simulink model "c2_non_lineare"  (R2021a)
settings: Solver=VariableStepAuto  StartTime=0.0  StopTime=10.0  RelTol=1e-3
values from neighbouring files (symbols this model uses):
  beta = 1.3    [c2.m]
  DD = 8    [c2.m]
  delta_1 = 3*10^4    (= 30000)    [c2.m]
  delta_2 = 0.2    [c2.m]
  delta_3 = 0.02    [c2.m]
  gamma_1 = 0.75    [c2.m]
  gamma_2 = 0.15    [c2.m]
  J = 20    [c2.m]
  phi = 0.04    [c2.m]
  RR_s = mu_s / G_0    [c2.m]
  u_e = (acos(-(gamma_2/gamma_1)*30*8e-4+1)+phi)/beta    [c2.m]
  x_1e = (delta_2 * x_2e + delta_3*x_2e^2) / delta_1    (= 0.0008)    [c2.m]
  x_2e = omega_e    (= 30)    [c2.m]
undefined symbols (not defined in the file or in its folder): NN, omega_d, omega_n, R_d
libraries: cstblocks x1
settings Model: Creator=lucac  LastModifiedBy=lucac

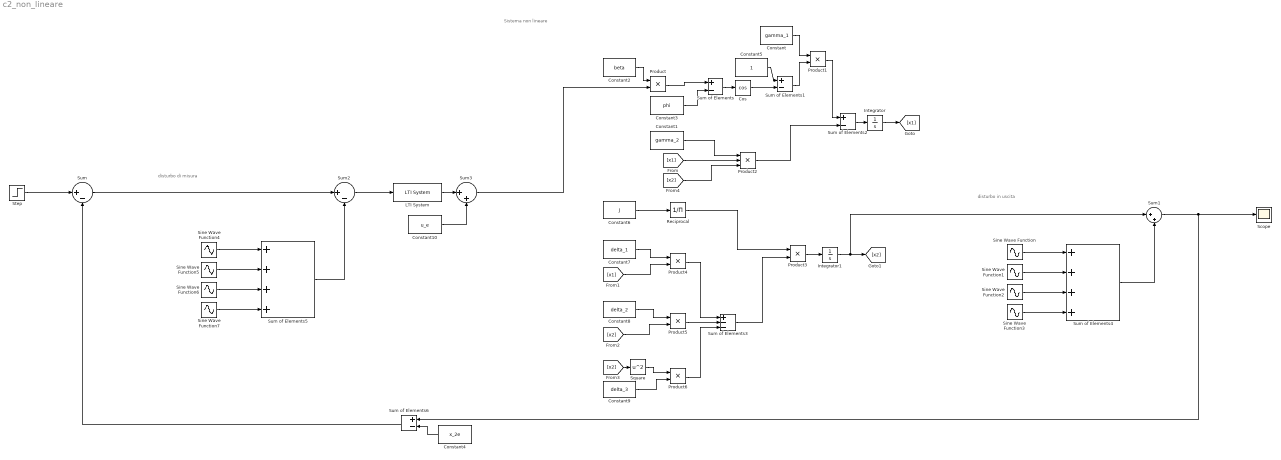
== system c2_non_lineare ==
  note: Sistema non lineare
  note: disturbo di misura
  note: disturbo in uscita
  Constant : Constant  Value=gamma_1
  Constant1 : Constant  Value=gamma_2
  Constant10 : Constant  Value=u_e
  Constant2 : Constant  Value=beta
  Constant3 : Constant  Value=phi
  Constant4 : Constant  Value=x_2e
  Constant5 : Constant
  Constant6 : Constant  Value=J
  Constant7 : Constant  Value=delta_1
  Constant8 : Constant  Value=delta_2
  Constant9 : Constant  Value=delta_3
  Cos : Trigonometry  Operator=cos
  Integrator : Integrator  InitialCondition=x_1e
  Integrator1 : Integrator  InitialCondition=x_2e
  LTI System : cstblocks/LTI System  sys=R_d*RR_s  IC=[]
  Product{,1,3..6} (6 alike) : Product
  Product2 : Product  Inputs=3
  Reciprocal : Product  Inputs=/
  Scope : Scope
  Sine Wave Function : Sin  TimeSource=Use external signal  Amplitude=DD  Frequency=omega_d  SampleTime=0
  Sine Wave Function1 : Sin  TimeSource=Use external signal  Amplitude=DD  Frequency=omega_d*2  SampleTime=0
  Sine Wave Function2 : Sin  TimeSource=Use external signal  Amplitude=DD  Frequency=omega_d*3  SampleTime=0
  Sine Wave Function3 : Sin  TimeSource=Use external signal  Amplitude=DD  Frequency=omega_d*4  SampleTime=0
  Sine Wave Function4 : Sin  TimeSource=Use external signal  Amplitude=NN  Frequency=omega_n  SampleTime=0
  Sine Wave Function5 : Sin  TimeSource=Use external signal  Amplitude=NN  Frequency=omega_n*2  SampleTime=0
  Sine Wave Function6 : Sin  TimeSource=Use external signal  Amplitude=NN  Frequency=omega_n*3  SampleTime=0
  Sine Wave Function7 : Sin  TimeSource=Use external signal  Amplitude=NN  Frequency=omega_n*4  SampleTime=0
  Square : Math  Operator=square  SaturateOnIntegerOverflow=on
  Step : Step  After=9  SampleTime=0
  Sum : Sum  Inputs=|+-
  Sum of Elements{,1..2,6} (4 alike) : Sum  Inputs=+-
  Sum of Elements3 : Sum  Inputs=+--
  Sum of Elements4 : Sum  Inputs=++++
  Sum of Elements5 : Sum  Inputs=++++
  Sum1 : Sum  Inputs=|++
  Sum2 : Sum  Inputs=|+-
  Sum3 : Sum  Inputs=|++
  wires:
  Constant2/1 -> Product/1
  Sum3/1 -> Product/2
  Product/1 -> Sum of Elements/1
  Constant3/1 -> Sum of Elements/2
  Sum of Elements/1 -> Cos/1
  Constant5/1 -> Sum of Elements1/1
  Cos/1 -> Sum of Elements1/2
  Sum of Elements1/1 -> Product1/2
  Constant/1 -> Product1/1
  Product1/1 -> Sum of Elements2/1
  Constant1/1 -> Product2/1
  Product2/1 -> Sum of Elements2/2
  Sum of Elements2/1 -> Integrator/1
  Constant6/1 -> Reciprocal/1
  Reciprocal/1 -> Product3/1
  Integrator/1 -> [x1]
  Constant7/1 -> Product4/1
  [x1] -> Product4/2
  Constant8/1 -> Product5/1
  [x2] -> Product5/2
  [x2] -> Square/1
  Square/1 -> Product6/1
  Constant9/1 -> Product6/2
  Product4/1 -> Sum of Elements3/1
  Product5/1 -> Sum of Elements3/2
  Product6/1 -> Sum of Elements3/3
  Sum of Elements3/1 -> Product3/2
  Product3/1 -> Integrator1/1
  Sine Wave Function/1 -> Sum of Elements4/1
  Sine Wave Function1/1 -> Sum of Elements4/2
  Sine Wave Function2/1 -> Sum of Elements4/3
  Sine Wave Function3/1 -> Sum of Elements4/4
  Integrator1/1 -> Sum1/1, [x2]
  Sum1/1 -> Sum of Elements6/1, Scope/1
  Sine Wave Function4/1 -> Sum of Elements5/1
  Sine Wave Function7/1 -> Sum of Elements5/4
  Sine Wave Function6/1 -> Sum of Elements5/3
  Sine Wave Function5/1 -> Sum of Elements5/2
  Sum/1 -> Sum2/1
  Sum2/1 -> LTI System/1
  LTI System/1 -> Sum3/1
  Constant10/1 -> Sum3/2
  [x1] -> Product2/2
  [x2] -> Product2/3
  Constant4/1 -> Sum of Elements6/2
  Sum of Elements6/1 -> Sum/2
  Step/1 -> Sum/1
  Sum of Elements5/1 -> Sum2/2
  Sum of Elements4/1 -> Sum1/2
